simulink model "RmtAPP"  (R2016b)
settings: Solver=VariableStepAuto  StartTime=0.0  StopTime=10.0  RelTol=1e-3
settings Model: Creator=bianxuyin  LastModifiedBy=bianxuyin

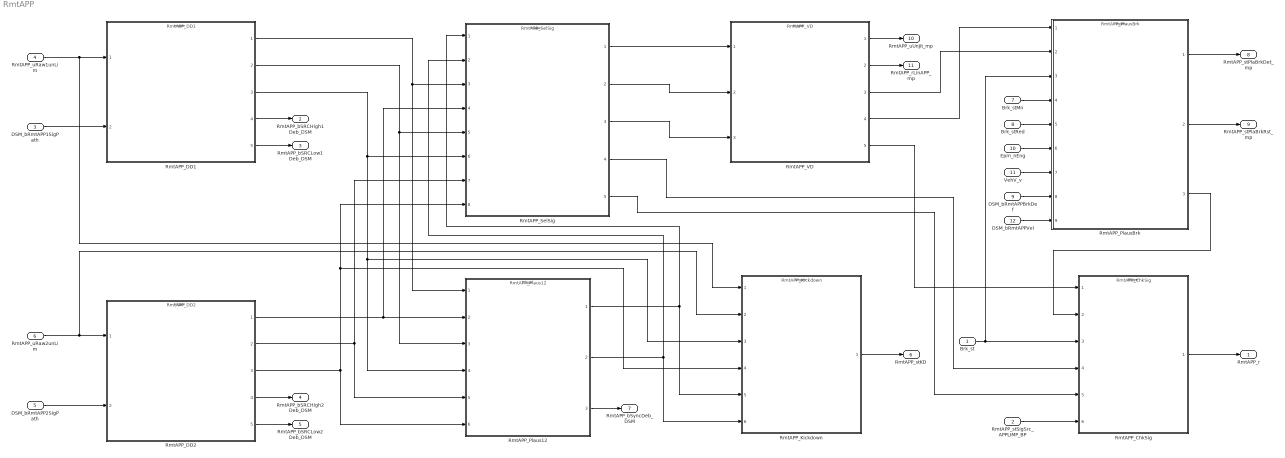
== system RmtAPP ==
  Brk_st : Inport  Description=Brake switch state  OutMin=0  OutMax=255  OutDataTypeStr=State_uint8
  RmtAPP_stSigSrc_APPLIMP_BP : Inport  Description=Substitute operation active, accelerator pedal sensor value and accelerator pedal sensor increase are limited  Port=2  OutMin=0  OutMax=1  OutDataTypeStr=boolean
  DSM_bRmtAPP1SigPath : Inport  Description=status of FId_APP1SigPath  Port=3  OutMin=0  OutMax=1  OutDataTypeStr=boolean
  RmtAPP_uRaw1unLim : Inport  Tag=mv  Description=Acceleration pedal sensor 1 unlimited raw value  Port=4  OutMin=0  OutMax=5000  OutDataTypeStr=Ad_mv
  DSM_bRmtAPP2SigPath : Inport  Description=status of FId_APP2SigPath  Port=5  OutMin=0  OutMax=1  OutDataTypeStr=boolean
  RmtAPP_uRaw2unLim : Inport  Tag=mv  Description=Acceleration pedal sensor 2 unlimited raw value  Port=6  OutMin=0  OutMax=5000  OutDataTypeStr=Ad_mv
  Brk_stMn : Inport  Description=Status of the main brake  Port=7  OutMin=0  OutMax=1  OutDataTypeStr=boolean
  Brk_stRed : Inport  Description=Status of the redundant break  Port=8  OutMin=0  OutMax=1  OutDataTypeStr=boolean
  DSM_bRmtAPPBrkDef : Inport  Description=status of FId_APPBrkDef  Port=9  OutMin=0  OutMax=1  OutDataTypeStr=boolean
  Epm_nEng : Inport  Tag=rpm  Description=Engine speed  Port=10  OutMin=0  OutMax=6000  OutDataTypeStr=EngSpeed_rpm
  VehV_v : Inport  Tag=km/h  Description=Vehicle speed  Port=11  OutMin=0  OutMax=250  OutDataTypeStr=VehSpeed_km_h
  DSM_bRmtAPPVel : Inport  Description=status of FId_APPVel  Port=12  OutMin=0  OutMax=1  OutDataTypeStr=boolean
  RmtAPP_ChkSig : ModelReference  ModelNameDialog=RmtAPP_ChkSig  SimulationMode=Normal  ModelReferenceVersion=1.13  TriggerPortName=function  TriggerPortTriggerType=function-call  TriggerPortStatesWhenEnabling=held
  RmtAPP_DD1 : ModelReference  ModelNameDialog=RmtAPP_DD1  SimulationMode=Normal  ModelReferenceVersion=1.7  TriggerPortName=function  TriggerPortTriggerType=function-call  TriggerPortStatesWhenEnabling=held
  RmtAPP_DD2 : ModelReference  ModelNameDialog=RmtAPP_DD2  SimulationMode=Normal  ModelReferenceVersion=1.5  TriggerPortName=function  TriggerPortTriggerType=function-call  TriggerPortStatesWhenEnabling=held
  RmtAPP_Kickdown : ModelReference  ModelNameDialog=RmtAPP_Kickdown  SimulationMode=Normal  ModelReferenceVersion=1.4  TriggerPortName=function  TriggerPortTriggerType=function-call  TriggerPortStatesWhenEnabling=held
  RmtAPP_Plaus12 : ModelReference  ModelNameDialog=RmtAPP_Plaus12  SimulationMode=Normal  ModelReferenceVersion=1.6  TriggerPortName=function  TriggerPortTriggerType=function-call  TriggerPortStatesWhenEnabling=held
  RmtAPP_PlausBrk : ModelReference  ModelNameDialog=RmtAPP_PlausBrk  SimulationMode=Normal  ModelReferenceVersion=1.8  TriggerPortName=function  TriggerPortTriggerType=function-call  TriggerPortStatesWhenEnabling=held
  RmtAPP_SelSig : ModelReference  ModelNameDialog=RmtAPP_SelSig  SimulationMode=Normal  ModelReferenceVersion=1.6  TriggerPortName=function  TriggerPortTriggerType=function-call  TriggerPortStatesWhenEnabling=held
  RmtAPP_VD : ModelReference  ModelNameDialog=RmtAPP_VD  SimulationMode=Normal  ModelReferenceVersion=1.12  TriggerPortName=function  TriggerPortTriggerType=function-call  TriggerPortStatesWhenEnabling=held
  RmtAPP_r : Outport  Tag=%  Description=Acceleration pedal sensor 1 value after fault handling  OutMin=0  OutMax=100  OutDataTypeStr=Accpedal_rate
  RmtAPP_bSRCHigh1Deb_DSM : Outport  Description=Status debounced SRC-High error Sensor 1  Port=2  OutMin=0  OutMax=1  OutDataTypeStr=boolean
  RmtAPP_bSRCLow1Deb_DSM : Outport  Description=Status debounced SRC-Low error Sensor 1  Port=3  OutMin=0  OutMax=1  OutDataTypeStr=boolean
  RmtAPP_bSRCHigh2Deb_DSM : Outport  Description=Status debounced SRC-High error Sensor 2  Port=4  OutMin=0  OutMax=1  OutDataTypeStr=boolean
  RmtAPP_bSRCLow2Deb_DSM : Outport  Description=Status debounced SRC-Low error Sensor 2  Port=5  OutMin=0  OutMax=1  OutDataTypeStr=boolean
  RmtAPP_stKD : Outport  Description=State of accelerator pedal kick down  Port=6  OutMin=0  OutMax=1  OutDataTypeStr=boolean
  RmtAPP_bSyncDeb_DSM : Outport  Description=Status debounced sync check finally defect  Port=7  OutMin=0  OutMax=1  OutDataTypeStr=boolean
  RmtAPP_stPlaBrkDet_mp : Outport  Description=State of detection plausibility with brake  Port=8  OutMin=0  OutMax=1  OutDataTypeStr=boolean
  RmtAPP_stPlaBrkRst_mp : Outport  Description=State of reset plausibility with brake  Port=9  OutMin=0  OutMax=1  OutDataTypeStr=boolean
  RmtAPP_uUnJit_mp : Outport  Tag=mv  Description=Acceleration pedal position unjittered value  Port=10  OutMin=0  OutMax=5000  OutDataTypeStr=Ad_mv
  RmtAPP_rLinAPP_mp : Outport  Tag=%  Description=Linearisation ratio of accelerator pedal  Port=11  OutMin=0  OutMax=100  OutDataTypeStr=Accpedal_rate
  wires:
  Brk_st/1 -> RmtAPP_ChkSig/3, RmtAPP_PlausBrk/3
  RmtAPP_stSigSrc_APPLIMP_BP/1 -> RmtAPP_ChkSig/6
  RmtAPP_Plaus12/1 -> RmtAPP_SelSig/1, RmtAPP_Kickdown/5
  RmtAPP_Plaus12/2 -> RmtAPP_Kickdown/6, RmtAPP_SelSig/2
  RmtAPP_DD1/3 -> RmtAPP_Plaus12/4, RmtAPP_Kickdown/3, RmtAPP_SelSig/6
  RmtAPP_DD1/1 -> RmtAPP_Plaus12/1, RmtAPP_SelSig/3
  RmtAPP_DD1/2 -> RmtAPP_Plaus12/3, RmtAPP_SelSig/5
  RmtAPP_DD2/1 -> RmtAPP_Plaus12/2, RmtAPP_SelSig/4
  RmtAPP_DD2/3 -> RmtAPP_Kickdown/4, RmtAPP_SelSig/8, RmtAPP_Plaus12/6
  RmtAPP_DD2/2 -> RmtAPP_SelSig/7, RmtAPP_Plaus12/5
  RmtAPP_ChkSig/1 -> RmtAPP_r/1
  RmtAPP_DD1/5 -> RmtAPP_bSRCLow1Deb_DSM/1
  RmtAPP_DD1/4 -> RmtAPP_bSRCHigh1Deb_DSM/1
  RmtAPP_DD2/4 -> RmtAPP_bSRCHigh2Deb_DSM/1
  RmtAPP_DD2/5 -> RmtAPP_bSRCLow2Deb_DSM/1
  RmtAPP_SelSig/1 -> RmtAPP_VD/1
  RmtAPP_SelSig/3 -> RmtAPP_VD/3
  RmtAPP_SelSig/2 -> RmtAPP_VD/2
  RmtAPP_SelSig/4 -> RmtAPP_ChkSig/4
  RmtAPP_SelSig/5 -> RmtAPP_ChkSig/5
  RmtAPP_Kickdown/1 -> RmtAPP_stKD/1
  RmtAPP_Plaus12/3 -> RmtAPP_bSyncDeb_DSM/1
  RmtAPP_PlausBrk/1 -> RmtAPP_stPlaBrkDet_mp/1
  RmtAPP_PlausBrk/2 -> RmtAPP_stPlaBrkRst_mp/1
  Brk_stMn/1 -> RmtAPP_PlausBrk/4
  DSM_bRmtAPPVel/1 -> RmtAPP_PlausBrk/9
  VehV_v/1 -> RmtAPP_PlausBrk/7
  DSM_bRmtAPPBrkDef/1 -> RmtAPP_PlausBrk/8
  Epm_nEng/1 -> RmtAPP_PlausBrk/6
  Brk_stRed/1 -> RmtAPP_PlausBrk/5
  RmtAPP_VD/5 -> RmtAPP_ChkSig/1
  RmtAPP_PlausBrk/3 -> RmtAPP_ChkSig/2
  RmtAPP_VD/4 -> RmtAPP_PlausBrk/1
  RmtAPP_VD/3 -> RmtAPP_PlausBrk/2
  RmtAPP_VD/1 -> RmtAPP_uUnJit_mp/1
  RmtAPP_VD/2 -> RmtAPP_rLinAPP_mp/1
  RmtAPP_uRaw1unLim/1 -> RmtAPP_Kickdown/1, RmtAPP_DD1/1
  DSM_bRmtAPP1SigPath/1 -> RmtAPP_DD1/2
  DSM_bRmtAPP2SigPath/1 -> RmtAPP_DD2/2
  RmtAPP_uRaw2unLim/1 -> RmtAPP_DD2/1, RmtAPP_Kickdown/2
